simulink model "tutorial28_dsp"  (R2025a)
settings: Solver=VariableStepAuto  StartTime=0.0  StopTime=10.0  RelTol=1e-3
libraries: simulink x1
settings Model: Creator=xing2  LastModifiedBy=xing2

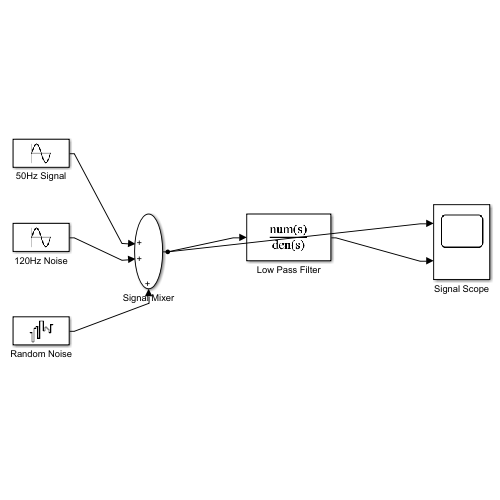
[thumbnail: Simulink's stored preview of the top-level diagram]
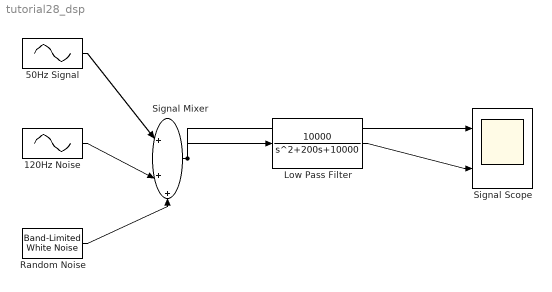
== system tutorial28_dsp ==
  120Hz Noise : Sin  Amplitude=0.5  Frequency=120  SampleTime=0
  50Hz Signal : Sin  Frequency=50  SampleTime=0
  Low Pass Filter : TransferFcn  Numerator=[10000]  Denominator=[1 200 10000]
  Random Noise : simulink/Sources/Band-Limited White Noise  Cov=[0.1]  Ts=0.1  seed=[23341]
  Signal Mixer : Sum  Inputs=|+++
  Signal Scope : Scope  NumInputPorts=2
  wires:
  50Hz Signal/1 -> Signal Mixer/1
  120Hz Noise/1 -> Signal Mixer/2
  Random Noise/1 -> Signal Mixer/3
  Signal Mixer/1 -> Low Pass Filter/1, Signal Scope/1
  Low Pass Filter/1 -> Signal Scope/2
